simulink model "untitled"  (R2017a)
settings: Solver=VariableStepAuto  StartTime=0.0  StopTime=4  MaxStep=0.01  RelTol=1e-4  EnableMultiTasking=on
libraries: simulink x2
settings Model: Creator=Shashi  LastModifiedBy=Shashi
settings DataIOCC: LimitDataPoints=on  SaveOutput=off  SaveTime=off
settings OptimizationCC: ExpressionDepthLimit=2147483647  LifeSpan=1
settings DebuggingCC: UnderspecifiedInitializationDetection=Classic  MergeDetectMultiDrivingBlocksExec=none  FcnCallInpInsideContextMsg=warning  AllowSymbolicDim=off  StateNameClashWarn=warning  SFUnexpectedBacktrackingDiag=warning  SFNoUnconditionalDefaultTransitionDiag=warning  SFExecutionAtInitializationDiag=none
settings GRTTargetCC: TargetLangStandard=C89/C90 (ANSI)  GeneratePreprocessorConditionals=Disable all  CombineOutputUpdateFcns=off  GRTInterface=on

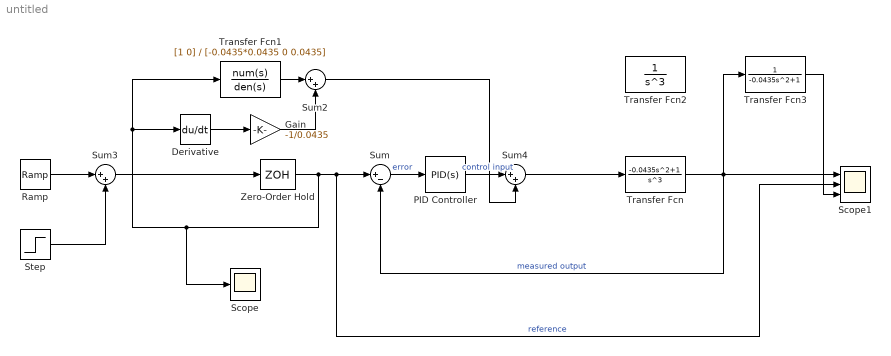
== system untitled ==
  Derivative : Derivative
  Gain : Gain  Gain=-1/0.0435
  PID Controller : simulink/Continuous/PID Controller  Controller=PID  TimeDomain=Continuous-time  SampleTime=-1  IntegratorMethod=Forward Euler  FilterMethod=Forward Euler  Form=Parallel  UseFilter=on  ControllerParametersSource=internal  P=-120769.985847755  I=-118097641.04215  D=4.97841756745276  N=8795.23735629613  InitialConditionSource=internal  InitialConditionForIntegrator=0  InitialConditionForFilter=0  ExternalReset=none  LimitOutput=off  UpperSaturationLimit=inf  LowerSaturationLimit=-inf  LinearizeAsGain=on  AntiWindupMode=none  Kb=1  TrackingMode=off  Kt=100  PParamMin=[]  PParamMax=[]  IParamMin=[]  IParamMax=[]  DParamMin=[]  DParamMax=[]  NParamMin=[]  NParamMax=[]  KbParamMin=[]  KbParamMax=[]  KtParamMin=[]  KtParamMax=[]  POutMin=[]  POutMax=[]  IOutMin=[]  IOutMax=[]  DOutMin=[]  DOutMax=[]  NOutMin=[]  NOutMax=[]  KbOutMin=[]  KbOutMax=[]  KtOutMin=[]  KtOutMax=[]  IntegratorOutMin=[]  IntegratorOutMax=[]  FilterOutMin=[]  FilterOutMax=[]  SumOutMin=[]  SumOutMax=[]  SumI1OutMin=[]  SumI1OutMax=[]  SumI2OutMin=[]  SumI2OutMax=[]  SumI3OutMin=[]  SumI3OutMax=[]  SumDOutMin=[]  SumDOutMax=[]  SaturationOutMin=[]  SaturationOutMax=[]  IntegratorContinuousStateAttributes=''  IntegratorStateMustResolveToSignalObject=off  IntegratorRTWStateStorageClass=Auto  FilterContinuousStateAttributes=''  FilterStateMustResolveToSignalObject=off  FilterRTWStateStorageClass=Auto  DifferentiatorICPrevScaledInput=0  DifferentiatorOutMin=[]  DifferentiatorOutMax=[]  InitialConditionSetting=State (most efficient)
  Ramp : simulink/Sources/Ramp  slope=16  start=1  X0=0
  Scope : Scope
  Scope1 : Scope  NumInputPorts=3
  Step : Step  After=8  SampleTime=0
  Sum : Sum  Inputs=|+-
  Sum2 : Sum  Inputs=|++
  Sum3 : Sum  Inputs=|++
  Sum4 : Sum  Inputs=|++
  Transfer Fcn : TransferFcn  Numerator=[-0.0435 0 1]  Denominator=[1 0 0 0]  ContinuousStateAttributes='plant'
  Transfer Fcn1 : TransferFcn  Numerator=[1 0]  Denominator=[-0.0435*0.0435 0 0.0435]  ContinuousStateAttributes='plan'
  Transfer Fcn2 : TransferFcn  Denominator=[1 0 0 0]  ContinuousStateAttributes='plant'
  Transfer Fcn3 : TransferFcn  Denominator=[-0.0435 0 1]  ContinuousStateAttributes='plant'
  Zero-Order Hold : ZeroOrderHold
  wires:
  Zero-Order Hold/1 -> Scope/1, Derivative/1, Transfer Fcn1/1, Scope1/2, Sum/1  "reference"
  Transfer Fcn/1 -> Transfer Fcn3/1, Scope1/1, Sum/2  "measured output"
  Transfer Fcn1/1 -> Sum2/1
  Derivative/1 -> Gain/1
  Gain/1 -> Sum2/2
  Ramp/1 -> Sum3/1
  Sum3/1 -> Zero-Order Hold/1
  Step/1 -> Sum3/2
  Sum/1 -> PID Controller/1  "error"
  PID Controller/1 -> Sum4/1  "control input"
  Sum4/1 -> Transfer Fcn/1
  Transfer Fcn3/1 -> Scope1/3
  Sum2/1 -> Sum4/2
